simulink model "DC_motor_with_PID"  (R2013b)
settings: Solver=ode45  StartTime=0.0  StopTime=20  MaxStep=0.1  RelTol=1e-3
values from neighbouring files (symbols this model uses):
  J = 1.66e-5    (= 1.66e-05)    [RunMotorSim.m]    (also in RunMotorSim_OpenLoop.m)
  KD = 1.33e-8    (= 1.33e-08)    [RunMotorSim.m]    (also in RunMotorSim_OpenLoop.m)
  KT = 7.5e-3    (= 0.0075)    [RunMotorSim.m]    (also in RunMotorSim_OpenLoop.m)
  pow = 1.88    [RunMotorSim.m]    (also in RunMotorSim_OpenLoop.m = 2)
undefined symbols (not defined in the file or in its folder): sigbuilder_block
libraries: simulink x3
settings Model: Creator=aberger  LastModifiedBy=aberger
settings DataIOCC: MaxDataPoints=100000

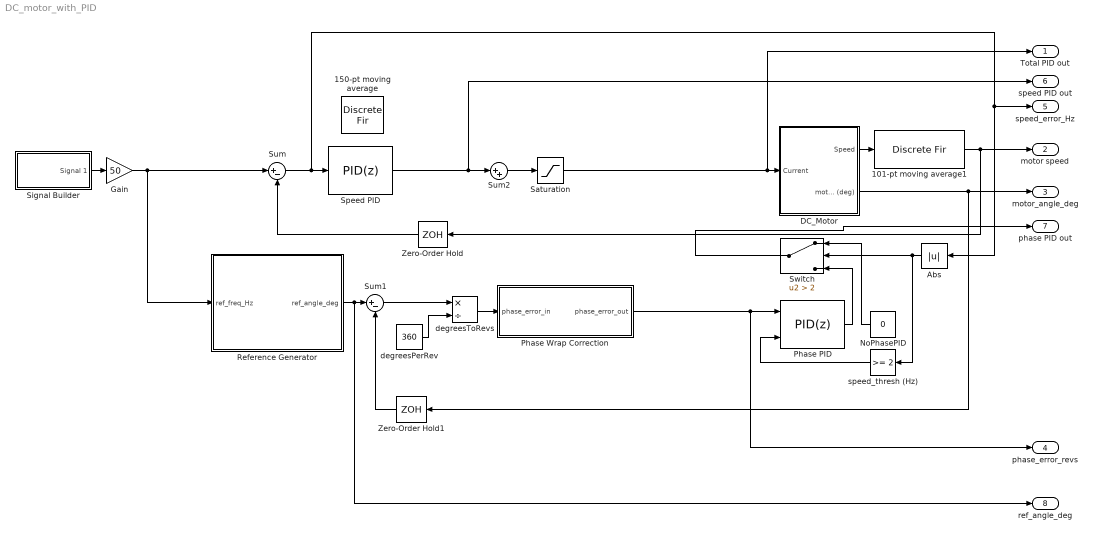
== system DC_motor_with_PID ==
  101-pt moving average1 : DiscreteFir  Coefficients="[0.00990099009900990\t0.00990099009900990\t0.00990099009900990\t0.00990099009900990\t0.00990099009900990\t0.00990099009900990\t0.00990099009900990\t0.00990099009900990\t0.00990099009900990\t0.00990099009900990\t0.00990099009900990\t0.00990099009900990\t0.00990099009900990\t0.00990099009900990\t0.00990099009900990\t0.00990099009900990\t0.00990099009900990\t0.00990099009900990\t0.00990099009900990\t0.00990099009900990\t0.00990099009900990\t0.00990099009900990\t0.00990099009900990\t0.00990099009900990\t0.00990099009900990\t0.00990099009900990\t0.00990099009900990\t0.00990099009900990\t0.00990099009900990\t0.00990099009900990\t0.00990099009900990\t0.00990099009900990\t0.00990099009900990\t0.00990099009900990\t0.00990099009900990\t0.00990099009900990\t0.00990099009900990\t0.00990099009900990\t0.00990099009900990\t0.00990099009900990\t0.00990099009900990\t0.00990099009900990\t0.00990099009900990\t0.00990099009900990\t0.00990099009900990\t0.00990099009900990\t0.00990099009900990\t0.00990099009900990\t0.00990099009900990\t0.00990099009900990\t0.00990099009900990\t0.00990099009900990\t0.00990099009900990\t0.00990099009900990\t0.00990099009900990\t0.00990099009900990\t0.00990099009900990\t0.00990099009900990\t0.00990099009900990\t0.00990099009900990\t0.00990099009900990\t0.00990099009900990\t0.00990099009900990\t0.00990099009900990\t0.00990099009900990\t0.00990099009900990\t0.00990099009900990\t0.00990099009900990\t0.00990099009900990\t0.00990099009900990\t0.00990099009900990\t0.00990099009900990\t0.00990099009900990\t0.00990099009900990\t0.00990099009900990\t0.00990099009900990\t0.00990099009900990\t0.00990099009900990\t0.00990099009900990\t0.00990099009900990\t0.00990099009900990\t0.00990099009900990\t0.00990099009900990\t0.00990099009900990\t0.00990099009900990\t0.00990099009900990\t0.00990099009900990\t0.00990099009900990\t0.00990099009900990\t0.00990099009900990\t0.00990099009900990\t0.00990099009900990\t0.00990099009900990\t0.00990099009900990\t0.00990099009900990\t0.00990099009900990\t0.00990099009900990\t0.00990099009900990\t0.00990099009900990\t0.00990099009900990\t0.00990099009900990]"
  150-pt moving average : DiscreteFir  Coefficients="[0.00666666666666667\t0.00666666666666667\t0.00666666666666667\t0.00666666666666667\t0.00666666666666667\t0.00666666666666667\t0.00666666666666667\t0.00666666666666667\t0.00666666666666667\t0.00666666666666667\t0.00666666666666667\t0.00666666666666667\t0.00666666666666667\t0.00666666666666667\t0.00666666666666667\t0.00666666666666667\t0.00666666666666667\t0.00666666666666667\t0.00666666666666667\t0.00666666666666667\t0.00666666666666667\t0.00666666666666667\t0.00666666666666667\t0.00666666666666667\t0.00666666666666667\t0.00666666666666667\t0.00666666666666667\t0.00666666666666667\t0.00666666666666667\t0.00666666666666667\t0.00666666666666667\t0.00666666666666667\t0.00666666666666667\t0.00666666666666667\t0.00666666666666667\t0.00666666666666667\t0.00666666666666667\t0.00666666666666667\t0.00666666666666667\t0.00666666666666667\t0.00666666666666667\t0.00666666666666667\t0.00666666666666667\t0.00666666666666667\t0.00666666666666667\t0.00666666666666667\t0.00666666666666667\t0.00666666666666667\t0.00666666666666667\t0.00666666666666667\t0.00666666666666667\t0.00666666666666667\t0.00666666666666667\t0.00666666666666667\t0.00666666666666667\t0.00666666666666667\t0.00666666666666667\t0.00666666666666667\t0.00666666666666667\t0.00666666666666667\t0.00666666666666667\t0.00666666666666667\t0.00666666666666667\t0.00666666666666667\t0.00666666666666667\t0.00666666666666667\t0.00666666666666667\t0.00666666666666667\t0.00666666666666667\t0.00666666666666667\t0.00666666666666667\t0.00666666666666667\t0.00666666666666667\t0.00666666666666667\t0.00666666666666667\t0.00666666666666667\t0.00666666666666667\t0.00666666666666667\t0.00666666666666667\t0.00666666666666667\t0.00666666666666667\t0.00666666666666667\t0.00666666666666667\t0.00666666666666667\t0.00666666666666667\t0.00666666666666667\t0.00666666666666667\t0.00666666666666667\t0.00666666666666667\t0.00666666666666667\t0.00666666666666667\t0.00666666666666667\t0.00666666666666667\t0.00666666666666667\t0.00666666666666667\t0.00666666666666667\t0.00666666666666667\t0.00666666666666667\t0.00666666666666667\t0.00666666666666667\t0.00666666666666667\t0.00666666666666667\t0.00666666666666667\t0.00666666666666667\t0.00666666666666667\t0.00666666666666667\t0.00666666666666667\t0.00666666666666667\t0.00666666666666667\t0.00666666666666667\t0.00666666666666667\t0.00666666666666667\t0.00666666666666667\t0.00666666666666667\t0.00666666666666667\t0.00666666666666667\t0.00666666666666667\t0.00666666666666667\t0.00666666666666667\t0.00666666666666667\t0.00666666666666667\t0.00666666666666667\t0.00666666666666667\t0.00666666666666667\t0.00666666666666667\t0.00666666666666667\t0.00666666666666667\t0.00666666666666667\t0.00666666666666667\t0.00666666666666667\t0.00666666666666667\t0.00666666666666667\t0.00666666666666667\t0.00666666666666667\t0.00666666666666667\t0.00666666666666667\t0.00666666666666667\t0.00666666666666667\t0.00666666666666667\t0.00666666666666667\t0.00666666666666667\t0.00666666666666667\t0.00666666666666667\t0.00666666666666667\t0.00666666666666667\t0.00666666666666667\t0.00666666666666667\t0.00666666666666667\t0.00666666666666667\t0.00666666666666667]"  SampleTime=.001
  Abs : Abs
  DC_Motor : Subsystem
  Gain : Gain  Gain=50
  NoPhasePID : Constant  Value=0
  Phase PID : simulink/Continuous/PID Controller  Controller=PID  TimeDomain=Discrete-time  SampleTime=.001  IntegratorMethod=Forward Euler  FilterMethod=Forward Euler  Form=Parallel  P=0.5  I=0.5  D=0.1  N=100  InitialConditionSource=internal  InitialConditionForIntegrator=0  InitialConditionForFilter=0  ExternalReset=level  LimitOutput=on  UpperSaturationLimit=1  LowerSaturationLimit=-1  LinearizeAsGain=on  AntiWindupMode=none  Kb=1  TrackingMode=off  Kt=1  PParamMin=[]  PParamMax=[]  IParamMin=[]  IParamMax=[]  DParamMin=[]  DParamMax=[]  NParamMin=[]  NParamMax=[]  KbParamMin=[]  KbParamMax=[]  KtParamMin=[]  KtParamMax=[]  POutMin=[]  POutMax=[]  IOutMin=[]  IOutMax=[]  DOutMin=[]  DOutMax=[]  NOutMin=[]  NOutMax=[]  KbOutMin=[]  KbOutMax=[]  KtOutMin=[]  KtOutMax=[]  IntegratorOutMin=[]  IntegratorOutMax=[]  FilterOutMin=[]  FilterOutMax=[]  SumOutMin=[]  SumOutMax=[]  SumI1OutMin=[]  SumI1OutMax=[]  SumI2OutMin=[]  SumI2OutMax=[]  SumI3OutMin=[]  SumI3OutMax=[]  SumDOutMin=[]  SumDOutMax=[]  SaturationOutMin=[]  SaturationOutMax=[]  IntegratorContinuousStateAttributes=''  IntegratorStateMustResolveToSignalObject=off  IntegratorRTWStateStorageClass=Auto  FilterContinuousStateAttributes=''  FilterStateMustResolveToSignalObject=off  FilterRTWStateStorageClass=Auto
  Phase Wrap Correction : Subsystem
  Reference Generator : Subsystem
  Saturation : Saturate  UpperLimit=1  LowerLimit=-1
  Signal Builder : Subsystem  Tag=STV Subsys  LoadFcn=sigbuilder_block('load');  StartFcn=sigbuilder_block('start');  StopFcn=sigbuilder_block('stop');  ClipboardFcn=sigbuilder_block('clipboard');  mask(Sigbuilder block){}
      mask help: Simulink:masks:SigbuilderBlock_MD
      mask init:
      | if ~strcmp(get_param(bdroot(gcbh),'SimulationStatus'),'stopped') tuvar = sigbuilder_block('maskInit'); end
      settings: CopyFcn=sigbuilder_block('copy');  DeleteFcn=sigbuilder_block('delete');  ModelCloseFcn=sigbuilder_block('modelClose');  PreSaveFcn=sigbuilder_block('preSave');  PauseFcn=sigbuilder_block('pause');  ContinueFcn=sigbuilder_block('continue');  NameChangeFcn=sigbuilder_block('namechange');  OpenFcn=sigbuilder_block('open',[437.25 199.5 550.5 399.75 ]);  CloseFcn=sigbuilder_block('close');
      mask Display: plot(0, 0, 100, 100,[2, 2, 32, 32, 2], [68, 8, 8, 68, 68],[32, 2], [38, 38], [32, 19, 2],[53, 60, 44], [32, 17, 17, 2],[16, 16, 31, 31]);txt = getActiveGroup(gcbh);text(2, 100, txt,'verticalAlignment', 'top');
  Speed PID : simulink/Continuous/PID Controller  Controller=PID  TimeDomain=Discrete-time  SampleTime=.001  IntegratorMethod=Forward Euler  FilterMethod=Forward Euler  Form=Parallel  P=.01  I=0  D=0  N=100  InitialConditionSource=internal  InitialConditionForIntegrator=0  InitialConditionForFilter=0  ExternalReset=none  LimitOutput=on  UpperSaturationLimit=1  LowerSaturationLimit=-1  LinearizeAsGain=on  AntiWindupMode=none  Kb=1  TrackingMode=off  Kt=1  PParamMin=[]  PParamMax=[]  IParamMin=[]  IParamMax=[]  DParamMin=[]  DParamMax=[]  NParamMin=[]  NParamMax=[]  KbParamMin=[]  KbParamMax=[]  KtParamMin=[]  KtParamMax=[]  POutMin=[]  POutMax=[]  IOutMin=[]  IOutMax=[]  DOutMin=[]  DOutMax=[]  NOutMin=[]  NOutMax=[]  KbOutMin=[]  KbOutMax=[]  KtOutMin=[]  KtOutMax=[]  IntegratorOutMin=[]  IntegratorOutMax=[]  FilterOutMin=[]  FilterOutMax=[]  SumOutMin=[]  SumOutMax=[]  SumI1OutMin=[]  SumI1OutMax=[]  SumI2OutMin=[]  SumI2OutMax=[]  SumI3OutMin=[]  SumI3OutMax=[]  SumDOutMin=[]  SumDOutMax=[]  SaturationOutMin=[]  SaturationOutMax=[]  IntegratorContinuousStateAttributes=''  IntegratorStateMustResolveToSignalObject=off  IntegratorRTWStateStorageClass=Auto  FilterContinuousStateAttributes=''  FilterStateMustResolveToSignalObject=off  FilterRTWStateStorageClass=Auto
  Sum : Sum  Inputs=|+-
  Sum1 : Sum  Inputs=|+-
  Sum2 : Sum  Inputs=|++
  Switch : Switch  Criteria=u2 > Threshold  Threshold=2
  Zero-Order Hold : ZeroOrderHold  SampleTime=.001
  Zero-Order Hold1 : ZeroOrderHold  SampleTime=.001
  degreesPerRev : Constant  Value=360
  degreesToRevs : Product  Inputs=*/
  speed_thresh (Hz) : simulink/Logic and Bit Operations/Compare To Constant  relop=>=  const=2  OutDataTypeStr=boolean
  Total PID out : Outport
  motor speed : Outport  Port=2
  motor_angle_deg : Outport  Port=3
  phase_error_revs : Outport  Port=4
  speed_error_Hz : Outport  Port=5
  speed PID out : Outport  Port=6
  phase PID out : Outport  Port=7
  ref_angle_deg : Outport  Port=8
  wires:
  Zero-Order Hold/1 -> Sum/2
  Reference Generator/1(ref_angle_deg) -> ref_angle_deg/1, Sum1/1
  DC_Motor/2(motor angle (deg)) -> motor_angle_deg/1, Zero-Order Hold1/1
  Sum2/1 -> Saturation/1
  Sum1/1 -> degreesToRevs/1
  degreesPerRev/1 -> degreesToRevs/2
  Zero-Order Hold1/1 -> Sum1/2
  degreesToRevs/1 -> Phase Wrap Correction/1(phase_error_in)
  Phase Wrap Correction/1(phase_error_out) -> Phase PID/1, phase_error_revs/1
  DC_Motor/1(Speed) -> 101-pt moving average1/1
  101-pt moving average1/1 -> motor speed/1, Zero-Order Hold/1
  Sum/1 -> speed_error_Hz/1, Abs/1, Speed PID/1
  Switch/1 -> phase PID out/1
  NoPhasePID/1 -> Switch/1
  Phase PID/1 -> Switch/3
  Abs/1 -> speed_thresh (Hz)/1, Switch/2
  speed_thresh (Hz)/1 -> Phase PID/2
  Signal Builder/1(Signal 1) -> Gain/1
  Gain/1 -> Reference Generator/1(ref_freq_Hz), Sum/1
  Saturation/1 -> Total PID out/1, DC_Motor/1(Current)
  Speed PID/1 -> speed PID out/1, Sum2/1

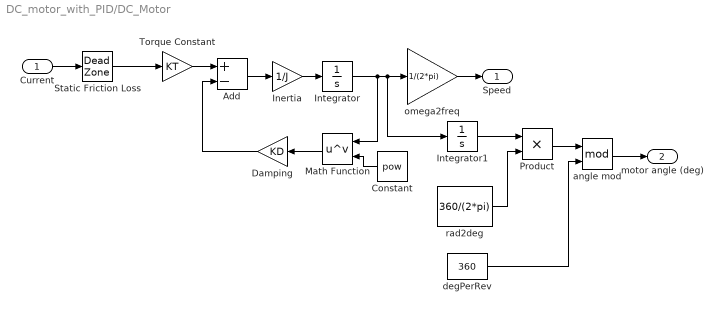
== system DC_motor_with_PID/DC_Motor ==
  Current : Inport
  Add : Sum  Inputs=+-
  Constant : Constant  Value=pow
  Damping : Gain  Gain=KD
  Inertia : Gain  Gain=1/J
  Integrator : Integrator
  Integrator1 : Integrator
  Math Function : Math  Operator=pow  SaturateOnIntegerOverflow=on
  Product : Product
  Static Friction Loss : DeadZone  LowerValue=-.05  UpperValue=.05  SaturateOnIntegerOverflow=on
  Torque Constant : Gain  Gain=KT
  angle mod : Math  Operator=mod  SaturateOnIntegerOverflow=on
  degPerRev : Constant  Value=360
  omega2freq : Gain  Gain=1/(2*pi)
  rad2deg : Constant  Value=360/(2*pi)
  Speed : Outport
  motor angle (deg) : Outport  Port=2
  wires:
  Add/1 -> Inertia/1
  Integrator/1 -> Math Function/1, Integrator1/1, omega2freq/1
  Torque Constant/1 -> Add/1
  Damping/1 -> Add/2
  Inertia/1 -> Integrator/1
  Current/1 -> Static Friction Loss/1
  Constant/1 -> Math Function/2
  Math Function/1 -> Damping/1
  omega2freq/1 -> Speed/1
  Integrator1/1 -> Product/1
  Product/1 -> angle mod/1
  rad2deg/1 -> Product/2
  degPerRev/1 -> angle mod/2
  Static Friction Loss/1 -> Torque Constant/1
  angle mod/1 -> motor angle (deg)/1

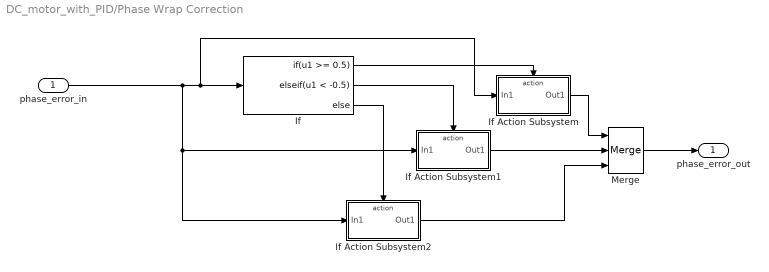
== system DC_motor_with_PID/Phase Wrap Correction ==
  phase_error_in : Inport
  If : If  IfExpression=u1 >= 0.5  ElseIfExpressions=u1 < -0.5
  If Action Subsystem : Subsystem  TreatAsAtomicUnit=on
  If Action Subsystem1 : Subsystem  TreatAsAtomicUnit=on
  If Action Subsystem2 : Subsystem  TreatAsAtomicUnit=on
  Merge : Merge  Inputs=3
  phase_error_out : Outport
  wires:
  If/1 -> If Action Subsystem/Action
  If Action Subsystem/1(Out1) -> Merge/1
  If Action Subsystem2/1(Out1) -> Merge/3
  phase_error_in/1 -> If/1, If Action Subsystem/1(In1), If Action Subsystem1/1(In1), If Action Subsystem2/1(In1)
  If/2 -> If Action Subsystem1/Action
  If/3 -> If Action Subsystem2/Action
  Merge/1 -> phase_error_out/1
  If Action Subsystem1/1(Out1) -> Merge/2

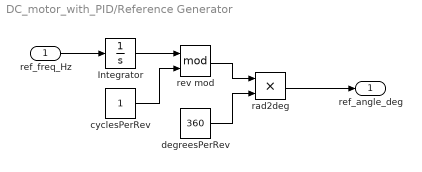
== system DC_motor_with_PID/Reference Generator ==
  ref_freq_Hz : Inport
  Integrator : Integrator
  cyclesPerRev : Constant
  degreesPerRev : Constant  Value=360
  rad2deg : Product
  rev mod : Math  Operator=mod  SaturateOnIntegerOverflow=on
  ref_angle_deg : Outport
  wires:
  cyclesPerRev/1 -> rev mod/2
  degreesPerRev/1 -> rad2deg/2
  Integrator/1 -> rev mod/1
  rev mod/1 -> rad2deg/1
  rad2deg/1 -> ref_angle_deg/1
  ref_freq_Hz/1 -> Integrator/1

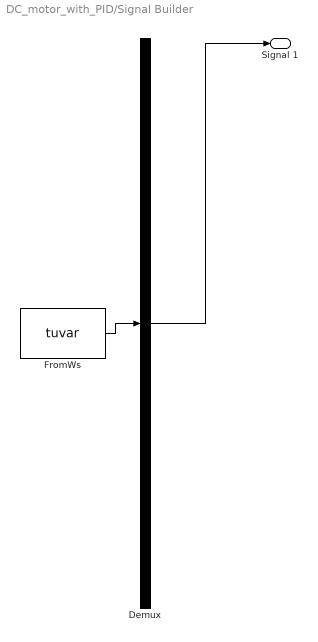
== system DC_motor_with_PID/Signal Builder ==
  Demux : Demux  Tag=STV Demux  Outputs=1
  FromWs : FromWorkspace  Tag=STV FromWs  VariableName=tuvar  SampleTime=0
      SigBuilderData=|
      | common.afterFinalStr = 'Extrapolate'
      | common.sampleTime = 0
      | dataSet.timeRange = [0 20]
      | dataSet.name = 'Group 1'
      | sbobj.Groups.Name = 'Group 1'
      | sbobj.Groups.Signals.Name = 'Signal 1'
      | sbobj.Groups.Signals.XData = [0 2.02 2.02 8 8 20]
      | sbobj.Groups.Signals.YData = [0 0 1 1 0.5 0.5]
      | sbobj.Groups.TimeRange = [0 20]
  Signal 1 : Outport  Tag=STV Outport
  wires:
  Demux/1 -> Signal 1/1
  FromWs/1 -> Demux/1

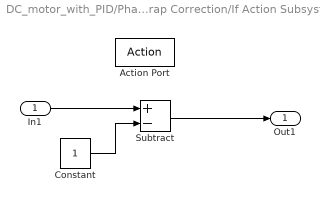
== system DC_motor_with_PID/Phase Wrap Correction/If Action Subsystem ==
  In1 : Inport
  Action Port : ActionPort  ActionType=then
  Constant : Constant
  Subtract : Sum  Inputs=+-
  Out1 : Outport
  wires:
  In1/1 -> Subtract/1
  Constant/1 -> Subtract/2
  Subtract/1 -> Out1/1

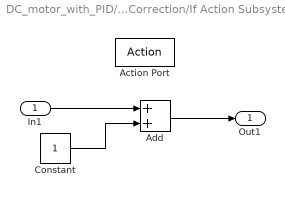
== system DC_motor_with_PID/Phase Wrap Correction/If Action Subsystem1 ==
  In1 : Inport
  Action Port : ActionPort  ActionType=elseif
  Add : Sum
  Constant : Constant
  Out1 : Outport
  wires:
  In1/1 -> Add/1
  Constant/1 -> Add/2
  Add/1 -> Out1/1

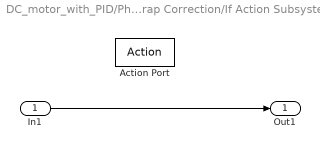
== system DC_motor_with_PID/Phase Wrap Correction/If Action Subsystem2 ==
  In1 : Inport
  Action Port : ActionPort  ActionType=else
  Out1 : Outport
  wires:
  In1/1 -> Out1/1
